simulink model "InjCrv_PiI1"  (R2016b)
settings: configuration reference "CodeGenConfigSet" (kept outside this file)
values from neighbouring files (symbols this model uses):
  InjCrv_phiPiI1Max_C = Calibration.Parameter    [init_InjCrv_PiI1.m]    (also in init_InjCrv_PiI1_SIL.m = Simulink.Parameter)
  InjCrv_qPiI1Max1_MAP = Calibration.Parameter    [init_InjCrv_PiI1.m]    (also in init_InjCrv_PiI1_SIL.m = Simulink.Parameter)
  InjCrv_qPiI1Max1_MAPX = Calibration.Parameter    [init_InjCrv_PiI1.m]    (also in init_InjCrv_PiI1_SIL.m = Simulink.Parameter)
  InjCrv_qPiI1Max1_MAPY = Calibration.Parameter    [init_InjCrv_PiI1.m]    (also in init_InjCrv_PiI1_SIL.m = Simulink.Parameter)
  InjCrv_stInjCharSetVal_C = Calibration.Parameter    [init_InjCrv_PiI1.m]    (also in init_InjCrv_PiI1_SIL.m = Simulink.Parameter)
  SigTst_phiPiI1_C = Calibration.Parameter    [init_InjCrv_PiI1.m]    (also in init_InjCrv_PiI1_SIL.m = Simulink.Parameter)
  SigTst_qPiI1_C = Calibration.Parameter    [init_InjCrv_PiI1.m]    (also in init_InjCrv_PiI1_SIL.m = Simulink.Parameter)
  SigTst_swtPiI1Phi_C = Calibration.Parameter    [init_InjCrv_PiI1.m]    (also in init_InjCrv_PiI1_SIL.m = Simulink.Parameter)
  SigTst_swtPiI1Q_C = Calibration.Parameter    [init_InjCrv_PiI1.m]    (also in init_InjCrv_PiI1_SIL.m = Simulink.Parameter)
  SigTst_swtPiI1Ti_C = Calibration.Parameter    [init_InjCrv_PiI1.m]    (also in init_InjCrv_PiI1_SIL.m = Simulink.Parameter)
  SigTst_tiPiI1_C = Calibration.Parameter    [init_InjCrv_PiI1.m]    (also in init_InjCrv_PiI1_SIL.m = Simulink.Parameter)
undefined symbols (not defined in the file or in its folder): Switch_conv
libraries: simulink x3
settings Model: Creator=Administrator  LastModifiedBy=mayongchao
settings ConfigSetRef: SourceLocation=Base Workspace

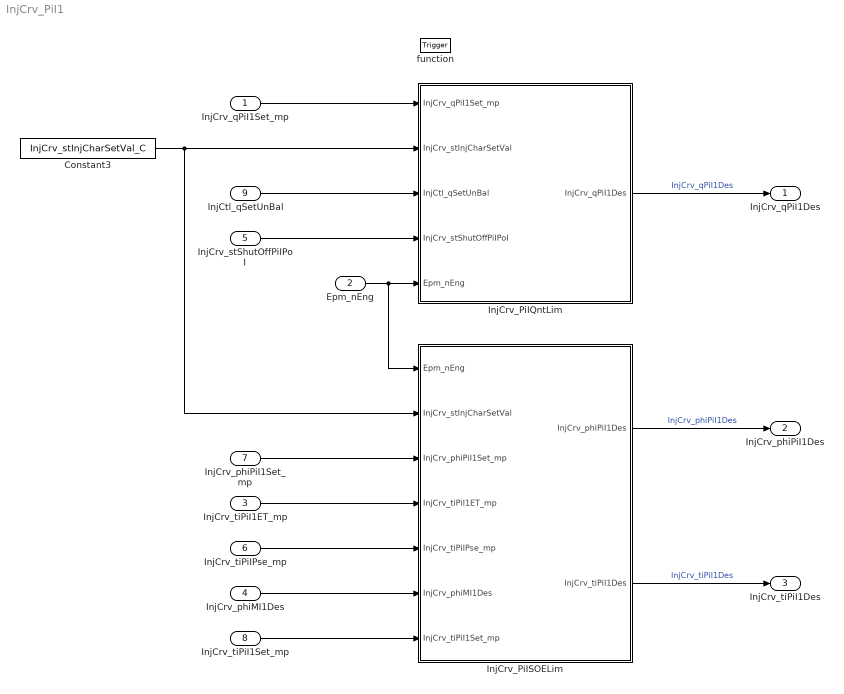
== system InjCrv_PiI1 ==
  InjCrv_qPiI1Set_mp : Inport  Tag=mg/hub  Description=Set PiI1 quantity  OutMin=-319  OutMax=319  OutDataTypeStr=FuelMass_mg_hub
  Epm_nEng : Inport  Tag=rpm  Description=Engine speed  Port=2  OutMin=0  OutMax=6000  OutDataTypeStr=EngSpeed_rpm
  InjCrv_tiPiI1ET_mp : Inport  Tag=us  Description=Estimated energizing time for PiI1  Port=3  OutMin=-13107  OutMax=13106  OutDataTypeStr=InjTime_us
  InjCrv_phiMI1Des : Inport  Tag=CA  Description=Desired reference angle for the start of MI1  Port=4  OutMin=-40  OutMax=40  OutDataTypeStr=Angle_CA
  InjCrv_stShutOffPiIPoI : Inport  Description=State of MI1 fuelMass too small  Port=5  OutMin=0  OutMax=1  OutDataTypeStr=boolean
  InjCrv_tiPiIPse_mp : Inport  Tag=us  Description=Minium injection interval between MI1 and PiI1  Port=6  OutMin=-13107  OutMax=13106  OutDataTypeStr=InjTime_us
  InjCrv_phiPiI1Set_mp : Inport  Tag=CA  Description=Set PiI1 start of energizing during starting time(phi)  Port=7  OutMin=-719  OutMax=719  OutDataTypeStr=Angle_CA
  InjCrv_tiPiI1Set_mp : Inport  Tag=us  Description=Set PiI1 start of energizing during starting time(ti)  Port=8  OutMin=-13107  OutMax=13106  OutDataTypeStr=InjTime_us
  InjCtl_qSetUnBal : Inport  Tag=mg/hub  Description=Current injection quantity  Port=9  OutMin=-319  OutMax=319  OutDataTypeStr=FuelMass_mg_hub
  function : TriggerPort  TriggerType=function-call  VariantControl=Variant
  Constant3 : Constant  Value=InjCrv_stInjCharSetVal_C
  InjCrv_PiIQntLim : Subsystem  RTWFcnName=InjCrv_PiIQntLim_Co  RTWFileName=InjCrv_PiI
      settings: RTWSystemCode=Nonreusable function  RTWFcnNameOpts=User specified  RTWFileNameOpts=User specified
  InjCrv_PiISOELim : Subsystem  RTWFcnName=InjCrv_PiISOELim_Co  RTWFileName=InjCrv_PiI
      settings: RTWSystemCode=Nonreusable function  RTWFcnNameOpts=User specified  RTWFileNameOpts=User specified
  InjCrv_qPiI1Des : Outport  Tag=mg/hub  Description=Desired PiI injection quantity  OutMin=-319  OutMax=319  OutDataTypeStr=FuelMass_mg_hub
  InjCrv_phiPiI1Des : Outport  Tag=CA  Description=Desired angular component for PiI1 start of energizing  Port=2  OutMin=-719  OutMax=719  OutDataTypeStr=Angle_CA
  InjCrv_tiPiI1Des : Outport  Tag=us  Description=Desired time component for PiI1 start of energizing  Port=3  OutMin=-13107  OutMax=13106  OutDataTypeStr=InjTime_us
  wires:
  InjCrv_PiIQntLim/1(InjCrv_qPiI1Des) -> InjCrv_qPiI1Des/1  "InjCrv_qPiI1Des"
  InjCrv_PiISOELim/1(InjCrv_phiPiI1Des) -> InjCrv_phiPiI1Des/1  "InjCrv_phiPiI1Des"
  InjCrv_PiISOELim/2(InjCrv_tiPiI1Des) -> InjCrv_tiPiI1Des/1  "InjCrv_tiPiI1Des"
  InjCrv_tiPiI1Set_mp/1 -> InjCrv_PiISOELim/7(InjCrv_tiPiI1Set_mp)
  InjCrv_phiMI1Des/1 -> InjCrv_PiISOELim/6(InjCrv_phiMI1Des)
  InjCrv_tiPiIPse_mp/1 -> InjCrv_PiISOELim/5(InjCrv_tiPiIPse_mp)
  InjCrv_tiPiI1ET_mp/1 -> InjCrv_PiISOELim/4(InjCrv_tiPiI1ET_mp)
  InjCrv_phiPiI1Set_mp/1 -> InjCrv_PiISOELim/3(InjCrv_phiPiI1Set_mp)
  InjCrv_qPiI1Set_mp/1 -> InjCrv_PiIQntLim/1(InjCrv_qPiI1Set_mp)
  Constant3/1 -> InjCrv_PiISOELim/2(InjCrv_stInjCharSetVal), InjCrv_PiIQntLim/2(InjCrv_stInjCharSetVal)
  InjCrv_stShutOffPiIPoI/1 -> InjCrv_PiIQntLim/4(InjCrv_stShutOffPiIPoI)
  InjCtl_qSetUnBal/1 -> InjCrv_PiIQntLim/3(InjCtl_qSetUnBal)
  Epm_nEng/1 -> InjCrv_PiIQntLim/5(Epm_nEng), InjCrv_PiISOELim/1(Epm_nEng)

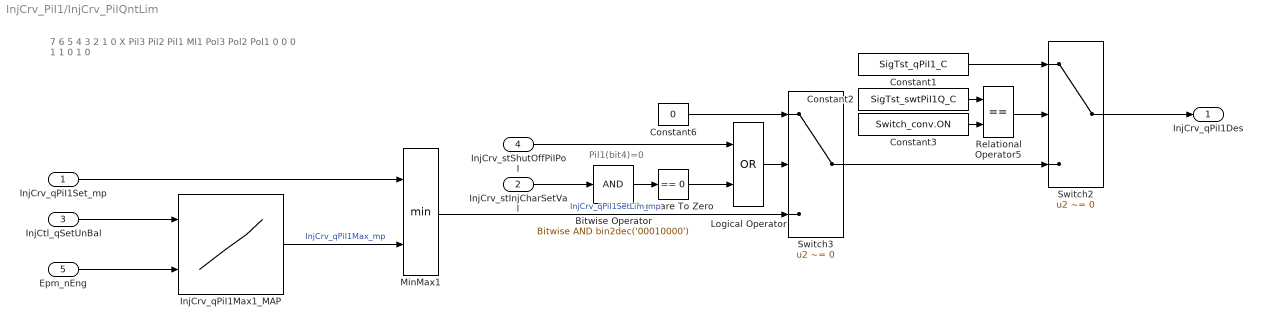
== system InjCrv_PiI1/InjCrv_PiIQntLim ==
  note: 7
      | 6
      | 5
      | 4
      | 3
      | 2
      | 1
      | 0
      |
      | X
      | Pil3
      | Pil2
      | Pil1
      | MI1
      | Pol3
      | Pol2
      | Pol1
      |
      | 0
      | 0
      | 0
      | 1
      | 1
      | 0
      | 1
      | 0
  note: Pil1(bit4)=0
  InjCrv_qPiI1Set_mp : Inport
  InjCrv_stInjCharSetVal : Inport  Port=2
  InjCtl_qSetUnBal : Inport  Port=3
  InjCrv_stShutOffPiIPoI : Inport  Port=4
  Epm_nEng : Inport  Port=5
  Bitwise Operator : simulink/Logic and Bit Operations/Bitwise Operator  logicop=AND  UseBitMask=on  BitMask=bin2dec('00010000')  BitMaskRealWorld=Stored Integer
  Compare To Zero : simulink/Logic and Bit Operations/Compare To Zero  relop===  OutDataTypeStr=boolean
  Constant1 : Constant  Value=SigTst_qPiI1_C
  Constant2 : Constant  RequirementInfo={'other' 'InjCrv_PiI_requirements.doc' '@Simulink_requirement_item_13' 'true' '手动设定预喷喷油量' '' } %GIDa_4c27cf4d_2e57_49b2_ad7f_0a4429589efc  Value=SigTst_swtPiI1Q_C
  Constant3 : Constant  RequirementInfo={'other' 'APP_requirements.doc' '@Simulink_requirement_item_25' 'true' '手动开关' '' } %GIDa_6dda4358_429e_4007_85ee_38592fc87e45  Value=Switch_conv.ON  OutDataTypeStr=Inherit: Inherit via back propagation
  Constant6 : Constant  Value=0  OutDataTypeStr=Inherit: Inherit via back propagation
  InjCrv_qPiI1Max1_MAP : Lookup_n-D  BreakpointsForDimension1=InjCrv_qPiI1Max1_MAPY  BreakpointsForDimension2=InjCrv_qPiI1Max1_MAPX  IndexSearchMethod=Linear search  BeginIndexSearchUsingPreviousIndexResult=on  Table=InjCrv_qPiI1Max1_MAP  ExtrapMethod=Clip  UseLastTableValue=on  InternalRulePriority=Speed  OutDataTypeStr=Inherit: Inherit via back propagation  SaturateOnIntegerOverflow=on
  Logical Operator : Logic  Operator=OR  AllPortsSameDT=off  OutDataTypeStr=boolean
  MinMax1 : MinMax  Inputs=2  InputSameDT=on
  Relational Operator5 : RelationalOperator  Operator===  OutDataTypeStr=boolean  RndMeth=Simplest  InputSameDT=on
  Switch2 : Switch  Criteria=u2 ~= 0  OutDataTypeStr=Inherit: Inherit via back propagation  RndMeth=Round  InputSameDT=on
  Switch3 : Switch  RequirementInfo={'other' 'InjCrv_PiI_requirements.doc' '@Simulink_requirement_item_19' 'true' '喷射状态控制' '' } %GIDa_9ab99534_129d_4f4b_95a5_156cec475e0c  Criteria=u2 ~= 0  OutDataTypeStr=Inherit: Inherit via back propagation  RndMeth=Round  InputSameDT=on
  InjCrv_qPiI1Des : Outport
  wires:
  InjCrv_stShutOffPiIPoI/1 -> Logical Operator/1
  Logical Operator/1 -> Switch3/2
  Constant3/1 -> Relational Operator5/2
  Switch3/1 -> Switch2/3
  Constant6/1 -> Switch3/1
  Bitwise Operator/1 -> Compare To Zero/1
  Compare To Zero/1 -> Logical Operator/2
  InjCrv_stInjCharSetVal/1 -> Bitwise Operator/1
  Switch2/1 -> InjCrv_qPiI1Des/1
  Constant1/1 -> Switch2/1
  Constant2/1 -> Relational Operator5/1
  MinMax1/1 -> Switch3/3  "InjCrv_qPiI1SetLim_mp"
  InjCrv_qPiI1Set_mp/1 -> MinMax1/1
  Relational Operator5/1 -> Switch2/2
  InjCrv_qPiI1Max1_MAP/1 -> MinMax1/2  "InjCrv_qPiI1Max_mp"
  InjCtl_qSetUnBal/1 -> InjCrv_qPiI1Max1_MAP/1
  Epm_nEng/1 -> InjCrv_qPiI1Max1_MAP/2

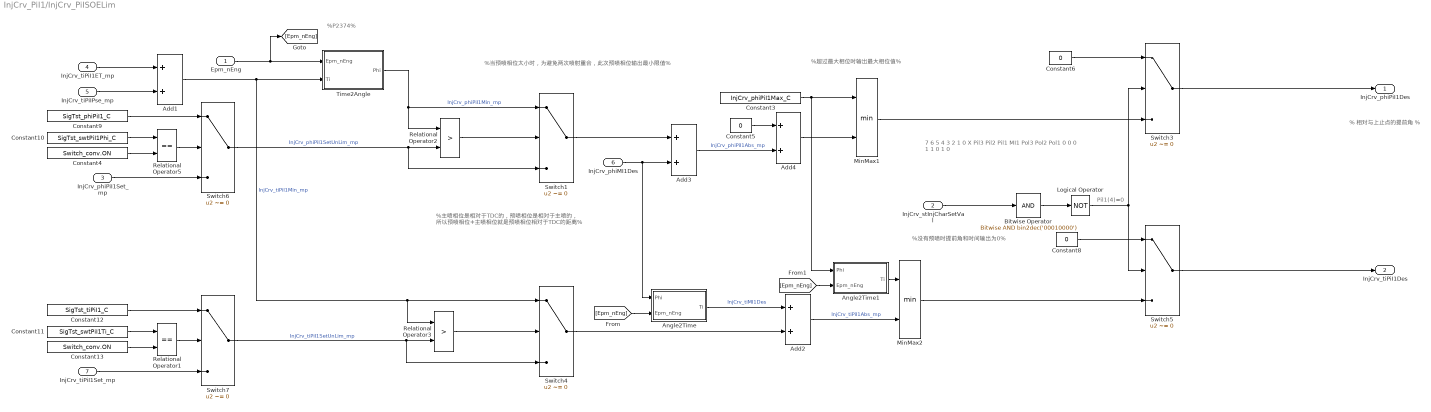
== system InjCrv_PiI1/InjCrv_PiISOELim ==
  note: % 相对与上止点的提前角 %
  note: 7
      | 6
      | 5
      | 4
      | 3
      | 2
      | 1
      | 0
      |
      | X
      | Pil3
      | Pil2
      | Pil1
      | MI1
      | Pol3
      | Pol2
      | Pol1
      |
      | 0
      | 0
      | 0
      | 1
      | 1
      | 0
      | 1
      | 0
  note: Pil1(4)=0
  note: %P2374%
  note: %主喷相位是相对于TDC的，预喷相位是相对于主喷的，
      | 所以预喷相位+主喷相位就是预喷相位相对于TDC的距离%
  note: %当预喷相位太小时，为避免两次喷射重合，此次预喷相位输出最小限值%
  note: %超过最大相位时输出最大相位值%
  note: %没有预喷时提前角和时间输出为0%
  Epm_nEng : Inport
  InjCrv_stInjCharSetVal : Inport  Port=2
  InjCrv_phiPiI1Set_mp : Inport  Port=3
  InjCrv_tiPiI1ET_mp : Inport  Port=4
  InjCrv_tiPiIPse_mp : Inport  Port=5
  InjCrv_phiMI1Des : Inport  Port=6
  InjCrv_tiPiI1Set_mp : Inport  Port=7
  Add1 : Sum  OutDataTypeStr=Inherit: Inherit via back propagation  RndMeth=Round  SaturateOnIntegerOverflow=on  InputSameDT=on
  Add2 : Sum  RndMeth=Round  SaturateOnIntegerOverflow=on  InputSameDT=on
  Add3 : Sum  RndMeth=Round  SaturateOnIntegerOverflow=on  InputSameDT=on
  Add4 : Sum  OutDataTypeStr=Inherit: Inherit via back propagation  RndMeth=Round  SaturateOnIntegerOverflow=on  InputSameDT=on
  Angle2Time : Subsystem
  Angle2Time1 : Subsystem
  Bitwise Operator : simulink/Logic and Bit Operations/Bitwise Operator  logicop=AND  UseBitMask=on  BitMask=bin2dec('00010000')  BitMaskRealWorld=Stored Integer
  Constant10 : Constant  Value=SigTst_swtPiI1Phi_C
  Constant11 : Constant  Value=SigTst_swtPiI1Ti_C
  Constant12 : Constant  Value=SigTst_tiPiI1_C
  Constant13 : Constant  RequirementInfo={'other' 'APP_requirements.doc' '@Simulink_requirement_item_25' 'true' '手动开关' '' } %GIDa_435216e9_b72a_48d6_afdb_10efbf826125  Value=Switch_conv.ON  OutDataTypeStr=Inherit: Inherit via back propagation
  Constant3 : Constant  Value=InjCrv_phiPiI1Max_C
  Constant4 : Constant  RequirementInfo={'other' 'APP_requirements.doc' '@Simulink_requirement_item_25' 'true' '手动开关' '' } %GIDa_5cc231b9_5b7a_4f4f_a147_e35632a03880  Value=Switch_conv.ON  OutDataTypeStr=Inherit: Inherit via back propagation
  Constant5 : Constant  Value=0  OutDataTypeStr=Inherit: Inherit via back propagation
  Constant6 : Constant  Value=0  OutDataTypeStr=Inherit: Inherit via back propagation
  Constant8 : Constant  Value=0  OutDataTypeStr=Inherit: Inherit via back propagation
  Constant9 : Constant  Value=SigTst_phiPiI1_C
  Logical Operator : Logic  Operator=NOT  AllPortsSameDT=off  OutDataTypeStr=boolean
  MinMax1 : MinMax  Inputs=2  RndMeth=Round  InputSameDT=on
  MinMax2 : MinMax  Inputs=2  RndMeth=Round  InputSameDT=on
  Relational Operator1 : RelationalOperator  Operator===  OutDataTypeStr=boolean  RndMeth=Simplest  InputSameDT=on
  Relational Operator2 : RelationalOperator  Operator=>  OutDataTypeStr=boolean  RndMeth=Nearest  InputSameDT=on
  Relational Operator3 : RelationalOperator  Operator=>  OutDataTypeStr=boolean  RndMeth=Nearest  InputSameDT=on
  Relational Operator5 : RelationalOperator  Operator===  OutDataTypeStr=boolean  RndMeth=Simplest  InputSameDT=on
  Switch1 : Switch  Criteria=u2 ~= 0  RndMeth=Round  InputSameDT=on
  Switch{3..7} (5 alike) : Switch  Criteria=u2 ~= 0  InputSameDT=on
  Time2Angle : Subsystem
  InjCrv_phiPiI1Des : Outport
  InjCrv_tiPiI1Des : Outport  Port=2
  wires:
  InjCrv_phiPiI1Set_mp/1 -> Switch6/3
  InjCrv_tiPiI1Set_mp/1 -> Switch7/3
  MinMax2/1 -> Switch5/3
  [Epm_nEng] -> Angle2Time1/2(Epm_nEng)
  [Epm_nEng] -> Angle2Time/2(Epm_nEng)
  Constant3/1 -> MinMax1/1, Angle2Time1/1(Phi)
  Angle2Time1/1(Ti) -> MinMax2/1
  Add2/1 -> MinMax2/2  "InjCrv_tiPiI1Abs_mp"
  Angle2Time/1(Ti) -> Add2/1  "InjCrv_tiMI1Des"
  Epm_nEng/1 -> Time2Angle/1(Epm_nEng), [Epm_nEng]
  Constant13/1 -> Relational Operator1/2
  Constant4/1 -> Relational Operator5/2
  Time2Angle/1(Phi) -> Relational Operator2/1, Switch1/1  "InjCrv_phiPiI1Min_mp"
  Logical Operator/1 -> Switch3/2, Switch5/2
  Bitwise Operator/1 -> Logical Operator/1
  Constant11/1 -> Relational Operator1/1
  Constant12/1 -> Switch7/1
  Constant10/1 -> Relational Operator5/1
  Constant9/1 -> Switch6/1
  Switch5/1 -> InjCrv_tiPiI1Des/1
  Constant8/1 -> Switch5/1
  Switch4/1 -> Add2/2
  Relational Operator3/1 -> Switch4/2
  Switch7/1 -> Relational Operator3/2, Switch4/3  "InjCrv_tiPiI1SetUnLim_mp"
  Add1/1 -> Time2Angle/2(Ti), Switch4/1, Relational Operator3/1  "InjCrv_tiPiI1Min_mp"
  Switch3/1 -> InjCrv_phiPiI1Des/1
  Constant6/1 -> Switch3/1
  InjCrv_stInjCharSetVal/1 -> Bitwise Operator/1
  MinMax1/1 -> Switch3/3
  Constant5/1 -> Add4/1
  Add4/1 -> MinMax1/2
  Add3/1 -> Add4/2  "InjCrv_phiPiI1Abs_mp"
  InjCrv_phiMI1Des/1 -> Add3/2, Angle2Time/1(Phi)
  Switch1/1 -> Add3/1
  Relational Operator2/1 -> Switch1/2
  Switch6/1 -> Relational Operator2/2, Switch1/3  "InjCrv_phiPiI1SetUnLim_mp"
  InjCrv_tiPiIPse_mp/1 -> Add1/2
  InjCrv_tiPiI1ET_mp/1 -> Add1/1
  Relational Operator5/1 -> Switch6/2
  Relational Operator1/1 -> Switch7/2

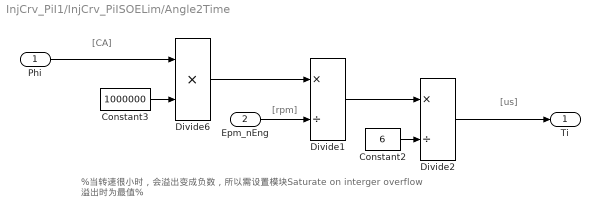
== system InjCrv_PiI1/InjCrv_PiISOELim/Angle2Time ==
  note: [CA]
  note: [rpm]
  note: [us]
  note: %当转速很小时，会溢出变成负数，所以需设置模块Saturate on interger overflow
      | 溢出时为最值%
  Phi : Inport
  Epm_nEng : Inport  Port=2
  Constant2 : Constant  Value=6  VectorParams1D=off  OutDataTypeStr=uint8
  Constant3 : Constant  Value=1000000  VectorParams1D=off  OutDataTypeStr=uint32
  Divide1 : Product  Inputs=*/  OutDataTypeStr=fixdt(1,32,3)  SaturateOnIntegerOverflow=on
  Divide2 : Product  Inputs=*/  OutDataTypeStr=Inherit: Inherit via back propagation  SaturateOnIntegerOverflow=on
  Divide6 : Product  Inputs=**  OutDataTypeStr=fixdt(1,32,3)  SaturateOnIntegerOverflow=on
  Ti : Outport
  wires:
  Constant3/1 -> Divide6/2
  Divide1/1 -> Divide2/1
  Constant2/1 -> Divide2/2
  Divide6/1 -> Divide1/1
  Phi/1 -> Divide6/1
  Epm_nEng/1 -> Divide1/2
  Divide2/1 -> Ti/1

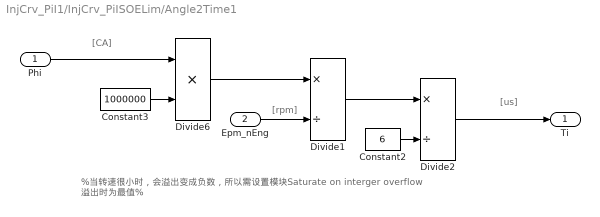
== system InjCrv_PiI1/InjCrv_PiISOELim/Angle2Time1 ==
  note: %当转速很小时，会溢出变成负数，所以需设置模块Saturate on interger overflow
      | 溢出时为最值%
  note: [us]
  note: [rpm]
  note: [CA]
  Phi : Inport
  Epm_nEng : Inport  Port=2
  Constant2 : Constant  Value=6  VectorParams1D=off  OutDataTypeStr=uint8
  Constant3 : Constant  Value=1000000  VectorParams1D=off  OutDataTypeStr=uint32
  Divide1 : Product  Inputs=*/  OutDataTypeStr=fixdt(1,32,3)  SaturateOnIntegerOverflow=on
  Divide2 : Product  Inputs=*/  OutDataTypeStr=Inherit: Inherit via back propagation  SaturateOnIntegerOverflow=on
  Divide6 : Product  Inputs=**  OutDataTypeStr=fixdt(1,32,3)  SaturateOnIntegerOverflow=on
  Ti : Outport
  wires:
  Divide2/1 -> Ti/1
  Epm_nEng/1 -> Divide1/2
  Phi/1 -> Divide6/1
  Divide6/1 -> Divide1/1
  Constant2/1 -> Divide2/2
  Divide1/1 -> Divide2/1
  Constant3/1 -> Divide6/2

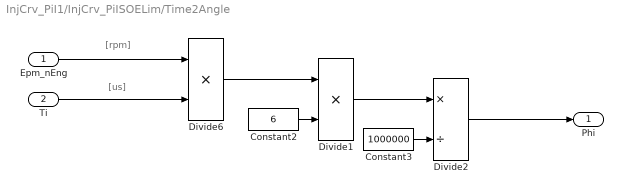
== system InjCrv_PiI1/InjCrv_PiISOELim/Time2Angle ==
  note: [rpm]
  note: [us]
  Epm_nEng : Inport
  Ti : Inport  Port=2
  Constant2 : Constant  Value=6  VectorParams1D=off  OutDataTypeStr=uint8
  Constant3 : Constant  Value=1000000  VectorParams1D=off  OutDataTypeStr=uint32
  Divide1 : Product  Inputs=**  OutDataTypeStr=fixdt(1,32,3)  SaturateOnIntegerOverflow=on
  Divide2 : Product  Inputs=*/  OutDataTypeStr=Inherit: Inherit via back propagation  SaturateOnIntegerOverflow=on
  Divide6 : Product  Inputs=**  OutDataTypeStr=fixdt(1,32,3)  SaturateOnIntegerOverflow=on
  Phi : Outport
  wires:
  Divide2/1 -> Phi/1
  Constant3/1 -> Divide2/2
  Divide1/1 -> Divide2/1
  Constant2/1 -> Divide1/2
  Divide6/1 -> Divide1/1
  Ti/1 -> Divide6/2
  Epm_nEng/1 -> Divide6/1
